simulink model "nonlinear"  (R2024a)
settings: Solver=VariableStepAuto  StartTime=0.0  StopTime=3  MaxStep=1e-3  RelTol=1e-3
values from neighbouring files (symbols this model uses):
  beta = m * lc    (= 40.0551)    [tester.m]
  f = 0    [tester.m]
  g = 9.81    [tester.m]
  J = (1/3)*m1*l^2 + m2*l^2    (= 62.720658)    [tester.m]
  M = 658.36    [tester.m]
  m = m1 + m2    (= 30.46)    [tester.m]
  x0 = [0;0;0.02;0]    [tester.m]
settings Model: Creator=eva  LastModifiedBy=eva

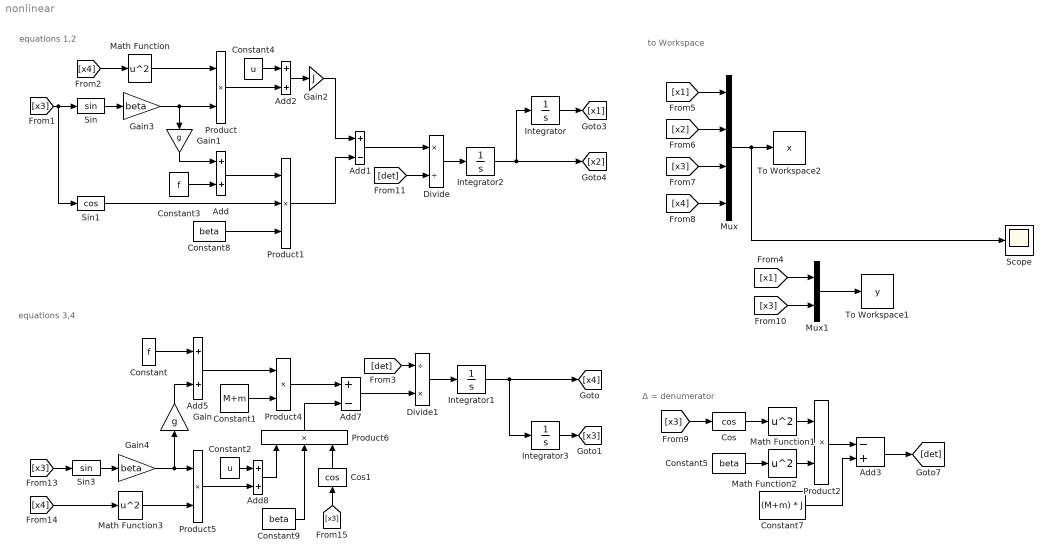
== system nonlinear ==
  note: equations 3,4
  note: equations 1,2
  note: to Workspace
  note: Δ = denumerator
  Add{,2,5,8} (4 alike) : Sum
  Add1 : Sum  Inputs=+-
  Add3 : Sum  Inputs=-+
  Add7 : Sum  Inputs=+-
  Constant : Constant  Value=f
  Constant1 : Constant  Value=M+m
  Constant2 : Constant  Value=u
  Constant3 : Constant  Value=f
  Constant4 : Constant  Value=u
  Constant5 : Constant  Value=beta
  Constant7 : Constant  Value=(M+m) * J
  Constant8 : Constant  Value=beta
  Constant9 : Constant  Value=beta
  Cos : Trigonometry  Operator=cos
  Cos1 : Trigonometry  Operator=cos
  Divide : Product  Inputs=*/
  Divide1 : Product  Inputs=/*
  Gain : Gain  Gain=g
  Gain1 : Gain  Gain=g
  Gain2 : Gain  Gain=J
  Gain3 : Gain  Gain=beta
  Gain4 : Gain  Gain=beta
  Integrator : Integrator  InitialCondition=x0(1)
  Integrator1 : Integrator  InitialCondition=x0(4)
  Integrator2 : Integrator  InitialCondition=x0(2)
  Integrator3 : Integrator  InitialCondition=x0(3)
  Math Function{,1..3} (4 alike) : Math  Operator=square
  Mux : Mux
  Mux1 : Mux  Inputs=2
  Product{,2,4..5} (4 alike) : Product
  Product1 : Product  Inputs=3
  Product6 : Product  Inputs=3
  Scope : Scope
  Sin : Trigonometry
  Sin1 : Trigonometry  Operator=cos
  Sin3 : Trigonometry
  To Workspace1 : ToWorkspace  VariableName=y  SaveFormat=Structure With Time  SampleTime=-1
  To Workspace2 : ToWorkspace  VariableName=x  SaveFormat=Structure With Time  SampleTime=-1
  wires:
  Mux/1 -> Scope/1, To Workspace2/1
  Integrator/1 -> [x1]
  Integrator2/1 -> [x2], Integrator/1
  Mux1/1 -> To Workspace1/1
  Divide/1 -> Integrator2/1
  [x3] -> Sin/1, Sin1/1
  Sin/1 -> Gain3/1
  [x4] -> Math Function/1
  Math Function/1 -> Product/1
  Gain3/1 -> Product/2, Gain1/1
  Product/1 -> Add2/2
  Constant4/1 -> Add2/1
  Add2/1 -> Gain2/1
  Constant3/1 -> Add/2
  Add/1 -> Product1/1
  Sin1/1 -> Product1/2
  Gain2/1 -> Add1/1
  Product1/1 -> Add1/2
  Gain1/1 -> Add/1
  Constant8/1 -> Product1/3
  [x1] -> Mux/1
  [x2] -> Mux/2
  [x3] -> Mux/3
  [x4] -> Mux/4
  [x3] -> Cos/1
  Cos/1 -> Math Function1/1
  Constant5/1 -> Math Function2/1
  Math Function1/1 -> Product2/1
  Math Function2/1 -> Product2/2
  Product2/1 -> Add3/1
  Constant7/1 -> Add3/2
  Add3/1 -> [det]
  Add1/1 -> Divide/1
  [det] -> Divide/2
  [det] -> Divide1/1
  Add5/1 -> Product4/1
  Product4/1 -> Add7/1
  Product5/1 -> Add8/2
  [x3] -> Sin3/1
  Sin3/1 -> Gain4/1
  [x4] -> Math Function3/1
  Add7/1 -> Divide1/2
  Constant1/1 -> Product4/2
  Constant2/1 -> Add8/1
  Product6/1 -> Add7/2
  [x3] -> Cos1/1
  Cos1/1 -> Product6/3
  Constant9/1 -> Product6/2
  Divide1/1 -> Integrator1/1
  Integrator1/1 -> [x4], Integrator3/1
  Integrator3/1 -> [x3]
  Add8/1 -> Product6/1
  [x1] -> Mux1/1
  [x3] -> Mux1/2
  Math Function3/1 -> Product5/2
  Gain4/1 -> Product5/1, Gain/1
  Constant/1 -> Add5/1
  Gain/1 -> Add5/2
